simulink model "real_time_distance_filter"  (R2020a)
settings: Solver=VariableStepAuto  StartTime=0.0  StopTime=1000  RelTol=1e-3
undefined symbols (not defined in the file): Discrete, sigbuilder_block, Time
libraries: simulink x2, ctrlSharedLib x1, dspstat3 x1
settings Model: Creator=ivory  LastModifiedBy=ivory

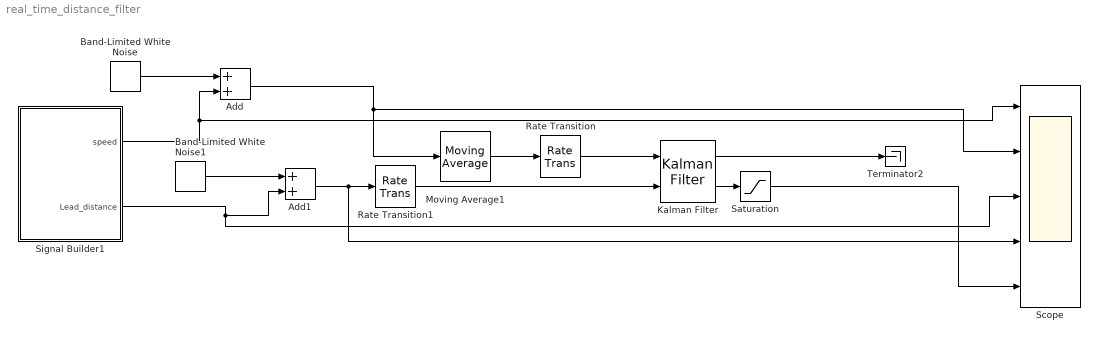
== system real_time_distance_filter ==
  Add : Sum
  Add1 : Sum
  Band-Limited White Noise : simulink/Sources/Band-Limited White Noise  Cov=0.001  Ts=0.1  seed=[23341]
  Band-Limited White Noise1 : simulink/Sources/Band-Limited White Noise  Cov=0.12  Ts=0.1  seed=[23341]
  Kalman Filter : ctrlSharedLib/Kalman Filter  TimeDomain=Discrete-Time  UseCurrentEstimator=on  ModelSource=LTI State-Space Variable  ModelSourceVariable=ss(-1, 1,1,0.2, 0.05)  A=0.95  B=1  C=1  D=0  NumberOfStates=1  NumberOfInputs=1  NumberOfOutputs=1  InitialEstimateSource=Dialog  X0=15  P0=10  UseK=off  UseGH=off  NumberOfProcessNoiseInputs=1  G=1  TimeInvariantG=on  H=0  TimeInvariantH=on  Q=0.76  TimeInvariantQ=on  R=0.001  TimeInvariantR=on  N=0  TimeInvariantN=on  AddInputPort=on  AddEnablePort=off  OutputEstimatedY=on  OutputP=off  Ts=-1
  Moving Average1 : dspstat3/Moving Average  Method=Sliding window  ForgettingFactorPort=off  SpecifyWindowLength=on  WindowLength=20  ForgettingFactor=0.9  SimulateUsing=Code generation
  Rate Transition : RateTransition  OutPortSampleTime=0.05
  Rate Transition1 : RateTransition  OutPortSampleTime=0.05
  Saturation : Saturate  UpperLimit=252  LowerLimit=0.0
  Scope : Scope  NumInputPorts=5
  Signal Builder1 : Subsystem  Tag=STV Subsys  LoadFcn=sigbuilder_block('load');  StartFcn=sigbuilder_block('start');  StopFcn=sigbuilder_block('stop');  ClipboardFcn=sigbuilder_block('clipboard');  mask(Sigbuilder block){tuvar=[0:10]}
      mask help: Simulink:masks:SigbuilderBlock_MD
      mask init:
      | if ~strcmp(get_param(bdroot(gcbh),'SimulationStatus'),'stopped') tuvar = sigbuilder_block('maskInit'); end
      settings: CopyFcn=sigbuilder_block('copy');  DeleteFcn=sigbuilder_block('delete');  ModelCloseFcn=sigbuilder_block('modelClose');  PreSaveFcn=sigbuilder_block('preSave');  PauseFcn=sigbuilder_block('pause');  ContinueFcn=sigbuilder_block('continue');  NameChangeFcn=sigbuilder_block('namechange');  OpenFcn=sigbuilder_block('open',[0 35.25 1440 567 ]);  CloseFcn=sigbuilder_block('close');
      mask Display: plot(0, 0, 100, 100,[2, 2, 32, 32, 2], [68, 8, 8, 68, 68],[32, 2], [38, 38], [32, 19, 2],[53, 60, 44], [32, 17, 17, 2],[16, 16, 31, 31]);txt = getActiveGroup(gcbh);text(2, 100, txt,'verticalAlignment', 'top');
  Terminator2 : Terminator
  wires:
  Saturation/1 -> Scope/5
  Kalman Filter/1 -> Terminator2/1
  Kalman Filter/2 -> Saturation/1
  Signal Builder1/1(speed) -> Add/2, Scope/1
  Signal Builder1/2(Lead_distance) -> Scope/3, Add1/2
  Add/1 -> Scope/2, Moving Average1/1
  Add1/1 -> Scope/4, Rate Transition1/1
  Moving Average1/1 -> Rate Transition/1
  Band-Limited White Noise/1 -> Add/1
  Band-Limited White Noise1/1 -> Add1/1
  Rate Transition/1 -> Kalman Filter/1
  Rate Transition1/1 -> Kalman Filter/2

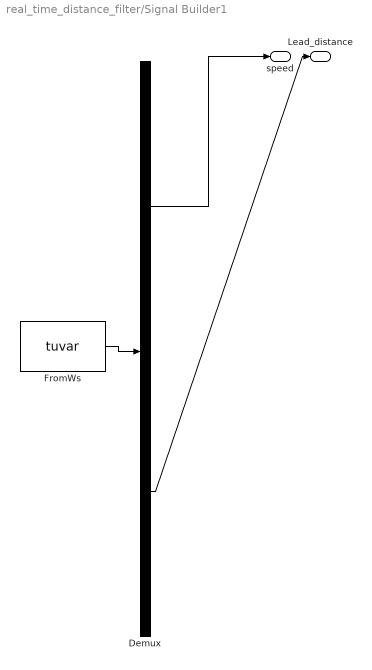
== system real_time_distance_filter/Signal Builder1 ==
  Demux : Demux  Tag=STV Demux  Outputs=2
      settings: DisplayOption=none
  FromWs : FromWorkspace  Tag=STV FromWs  VariableName=tuvar
      SigBuilderData=|
      | common.afterFinalStr = 'Extrapolate'
      | common.sampleTime = 0
      | dataSet.timeRange = [0 1000]
      | dataSet.name = 'Group 1'
      | sbobj.Groups.Name = 'Group 1'
      | sbobj.Groups.Signals(1).Name = 'speed'
      | sbobj.Groups.Signals(1).XData = [0 0.0175309181213 0.0361220836639 0.055948972702 0.0736720561981 0.241894006729 0.442004919052 0.642072916031 0.841996908188 1.04228997231 1.24200797081 1.44191408157 ... (5580 elements, 1x5580)]
      | sbobj.Groups.Signals(1).YData = [0 0 0 0 0 0 0 0 0 0 0 0 ... (5580 elements, 1x5580)]
      | sbobj.Groups.Signals(2).Name = 'Lead_distance'
      | sbobj.Groups.Signals(2).XData = [0 0.0175309181213 0.0361220836639 0.055948972702 0.0736720561981 0.241894006729 0.442004919052 0.642072916031 0.841996908188 1.04228997231 1.24200797081 1.44191408157 ... (5580 elements, 1x5580)]
      | sbobj.Groups.Signals(2).YData = [252 252 252 252 252 252 252 252 252 252 252 252 ... (5580 elements, 1x5580)]
      | sbobj.Groups.TimeRange = [0 1000]
  speed : Outport  Tag=STV Outport
  Lead_distance : Outport  Tag=STV Outport  Port=2
  wires:
  FromWs/1 -> Demux/1
  Demux/1 -> speed/1
  Demux/2 -> Lead_distance/1
